simulink model "modelo_motor_P2_LUT"  (R2021b)
settings: Solver=VariableStepAuto  StartTime=0.0  StopTime=T_end  RelTol=1e-3
values from neighbouring files (symbols this model uses):
  Gz = c2d(G,Tm)    [lanza_P2.m]
  k = 3.6    [lanza_P2.m]
  k_nl = 3.6    [lanza_P2.m]
  m = 3    [lanza_P2.m]
  Tm = 0.01    [lanza_P2.m]
  Vel_sat = 9.5    [lanza_P2.m]
  Volt = [0.25 0.5 0.75 1 2 3 4 5 6 7 8 9]    [lanza_P2.m]
  Volt_dead = 1    [lanza_P2.m]
libraries: cstblocks x3, dspsrcs4 x2
settings Model: Creator=jvalls  LastModifiedBy=jgragia
settings SolverCC: AlgebraicLoopSolver=TrustRegion
settings DataIOCC: ReturnWorkspaceOutputs=off
settings OptimizationCC: LifeSpan=inf
settings DebuggingCC: SFExecutionAtInitializationDiag=none  SFMachineParentedDataDiag=warning  ArithmeticOperatorsInVariantConditions=warning
settings SFSimCC: SimUseLocalCustomCode=off  CustomCodeUndefinedFunction=UseInterfaceOnly
settings RTWCC: RTWUseLocalCustomCode=off
settings CodeAppCC: StateflowObjectComments=on

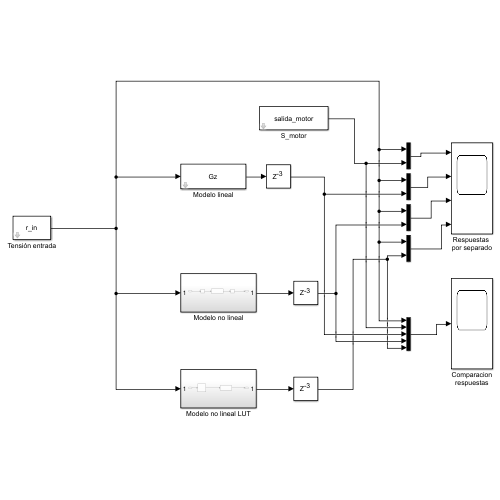
[thumbnail: Simulink's stored preview of the top-level diagram]
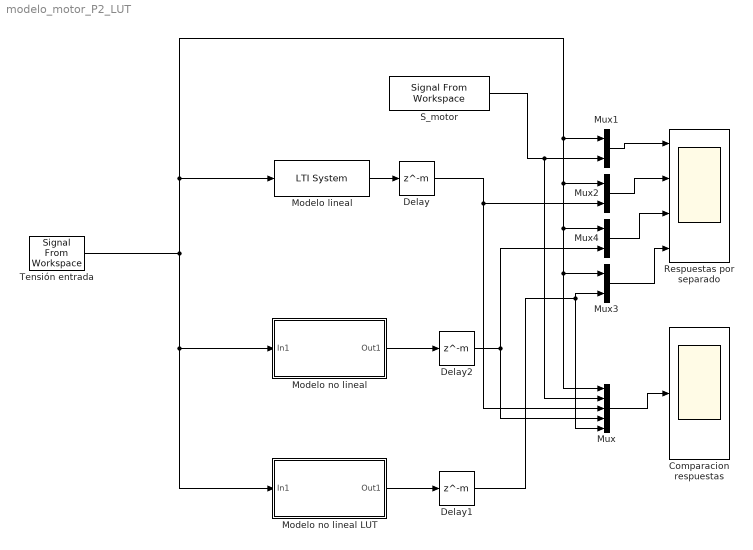
== system modelo_motor_P2_LUT ==
  Comparacion respuestas : Scope
  Delay : Delay  DelayLength=m  InitialCondition=0
  Delay1 : Delay  DelayLength=m  InitialCondition=0
  Delay2 : Delay  DelayLength=m  InitialCondition=0
  Modelo lineal : cstblocks/LTI System  sys=Gz  IC=[]
  Modelo no lineal : Subsystem
  Modelo no lineal LUT : Subsystem
  Mux : Mux  Inputs=5
  Mux{1..4} (4 alike) : Mux  Inputs=2
  Respuestas por separado : Scope  NumInputPorts=4
  S_motor : dspsrcs4/Signal From Workspace  X=salida_motor  Ts=Tm  nsamps=1  OutputAfterFinalValue=Setting to zero  ignoreOrWarnInputAndFrameLengths=off  OutputFrames=off
  Tensión entrada : dspsrcs4/Signal From Workspace  X=r_in  Ts=Tm  nsamps=1  OutputAfterFinalValue=Setting to zero  ignoreOrWarnInputAndFrameLengths=off  OutputFrames=off
  wires:
  Modelo lineal/1 -> Delay/1
  S_motor/1 -> Mux1/2, Mux/2
  Mux/1 -> Comparacion respuestas/1
  Mux1/1 -> Respuestas por separado/1
  Mux2/1 -> Respuestas por separado/2
  Mux3/1 -> Respuestas por separado/4
  Modelo no lineal LUT/1(Out1) -> Delay1/1
  Delay/1 -> Mux2/2, Mux/3
  Delay1/1 -> Mux/5, Mux3/2
  Tensión entrada/1 -> Modelo no lineal/1(In1), Modelo no lineal LUT/1(In1), Modelo lineal/1, Mux1/1, Mux2/1, Mux4/1, Mux3/1, Mux/1
  Modelo no lineal/1(Out1) -> Delay2/1
  Delay2/1 -> Mux4/2, Mux/4
  Mux4/1 -> Respuestas por separado/3

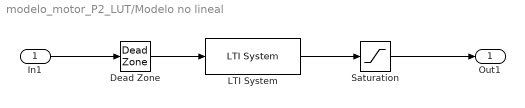
== system modelo_motor_P2_LUT/Modelo no lineal ==
  In1 : Inport
  "Dead Zone " : DeadZone  LowerValue=-Volt_dead  UpperValue=Volt_dead
  "LTI System " : cstblocks/LTI System  sys=Gz*k_nl  IC=[]
  "Saturation " : Saturate  UpperLimit=Vel_sat  LowerLimit=-Vel_sat
  Out1 : Outport
  wires:
  "LTI System "/1 -> "Saturation "/1
  In1/1 -> "Dead Zone "/1
  "Saturation "/1 -> Out1/1
  "Dead Zone "/1 -> "LTI System "/1

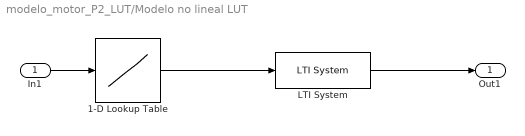
== system modelo_motor_P2_LUT/Modelo no lineal LUT ==
  In1 : Inport
  "1-D Lookup Table " : Lookup_n-D  NumberOfTableDimensions=1  BreakpointsForDimension1=[Volt 100]  Table=[Vel Vel(end)]  InternalRulePriority=Speed  RndMeth=Simplest  InputSameDT=on
  "LTI System " : cstblocks/LTI System  sys=Gz/k  IC=[]
  Out1 : Outport
  wires:
  In1/1 -> "1-D Lookup Table "/1
  "LTI System "/1 -> Out1/1
  "1-D Lookup Table "/1 -> "LTI System "/1
